simulink model "Inverter_2_"  (R2020a)
settings: Solver=VariableStepAuto  StartTime=0.0  StopTime=0.0335  RelTol=1e-3
libraries: powerlib x10
settings Model: Creator=Naeem Mohammad  LastModifiedBy=Naeem Mohammad

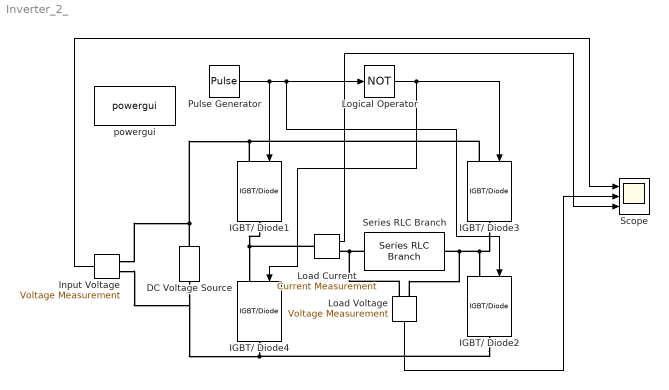
== system Inverter_2_ ==
  DC Voltage Source : powerlib/Electrical Sources/DC Voltage Source  Amplitude=48  Measurements=None
  IGBT/ Diode{1..4} (4 alike) : powerlib/Power Electronics/IGBT//Diode  Ron=1e-3  Rs=1e5  Cs=inf  Measurements=off
  Input Voltage : powerlib/Measurements/Voltage Measurement  PhasorSimulation=off  OutputType=Complex  PSBequivalent=0
  Load Current : powerlib/Measurements/Current Measurement  PhasorSimulation=off  OutputType=Complex  PSBequivalent=0
  Load Voltage : powerlib/Measurements/Voltage Measurement  PhasorSimulation=off  OutputType=Complex  PSBequivalent=0
  Logical Operator : Logic  Operator=NOT  AllPortsSameDT=off  OutDataTypeStr=boolean
  Pulse Generator : DiscretePulseGenerator  PulseType=Time based  Period=0.0167  PulseWidth=50
  Scope : Scope  NumInputPorts=3
  Series RLC Branch : powerlib/Elements/Series RLC Branch  LConnTagsString=__new0  RConnTagsString=__new0  BranchType=R  Resistance=5  Inductance=10e-4  SetiL0=off  InitialCurrent=0  Capacitance=1e-6  Setx0=off  InitialVoltage=0  Measurements=None
  powergui : powerlib/powergui  Priority=1  SimulationMode=Continuous  SampleTime=50e-6  frequency=60  Iterations=50  frequencyindice=0  Pbase=100e6  ErrMax=1e-4  UnitsV=kV  UnitsW=MW  buscounter=0  FunctionMessages=off  echomessages=off  EnableUseOfTLC=off  CurrentSourceSwitches=off  DisableSnubberDevices=off  DisableRonSwitches=off  DisableVfSwitches=off  DisplayEquations=off  AutomaticDiscreteSolvers=off  SolverType=Tustin/Backward Euler (TBE)  Interpol=off  ExternalGateDelay=off  methode=off  Ts=100  x0status=blocks  SPID=on  SwTol=0  HookPort=off  NonlinearTolerance=1e-4  nMaxIteration=100  ContinueOnMaxIteration=off  RestoreLinks=warning  ResistiveCurrentMeasurement=off  Frange=[0:2:500]  Ylog=off  Xlog=on  ShowGrid=off  save=off  variable=ZData  structure=0  ZoomFFT=off  StartTime=0.0  cycles=1  DisplayStyle=1  fundamental=60  FreqAxis=off  MaxFrequency=1000  frequencyindicesteady=1  RmsSteady=1  display=off
  wires:
  Load Current/1 -> Scope/3
  Logical Operator/1 -> IGBT/ Diode3/1, IGBT/ Diode4/1
  Pulse Generator/1 -> IGBT/ Diode1/1, IGBT/ Diode2/1, Logical Operator/1
  Load Voltage/1 -> Scope/2
  Input Voltage/1 -> Scope/1
  connections:
  Series RLC Branch/LConn1 -- Load Voltage/LConn1 -- Load Current/RConn1
  IGBT/ Diode3/RConn1 -- Load Voltage/LConn2 -- Series RLC Branch/RConn1 -- IGBT/ Diode2/LConn1
  DC Voltage Source/RConn1 -- Input Voltage/LConn1 -- IGBT/ Diode1/LConn1 -- IGBT/ Diode3/LConn1
  IGBT/ Diode2/RConn1 -- Input Voltage/LConn2 -- DC Voltage Source/LConn1 -- IGBT/ Diode4/RConn1
  IGBT/ Diode1/RConn1 -- Load Current/LConn1 -- IGBT/ Diode4/LConn1
